simulink model "FEEDER_MODEL"  (R2024b)
settings: Solver=ode23t  StartTime=0.0  StopTime=2.4  RelTol=1e-3
libraries: spsFirstOrderFilterLib x42, spsThreePhaseVIMeasurementLib x7, spsThreePhaseDynamicLoadLib x4, spsDistributedParametersLineLib x4, spsPower3phInstantaneousLib x3, spsThreePhaseSourceLib x2, spsThreePhaseTransformerTwoWindingsLib x2, spspowerguiLib x1
(part 2 of 2)

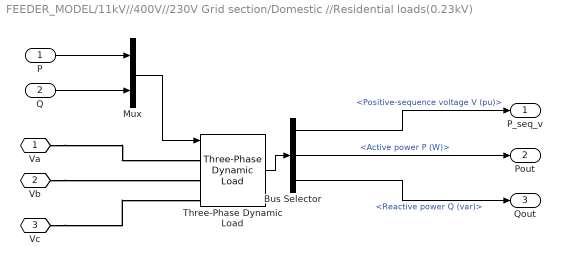
== system FEEDER_MODEL/11kV//400V//230V Grid section/Domestic //Residential loads(0.23kV) ==
  P : Inport
  Q : Inport  Port=2
  Bus Selector : BusSelector  OutputSignals=Positive-sequence voltage V (pu),Active power P (W),Reactive power Q (var)
  Mux : Mux  Inputs=2
  Three-Phase Dynamic Load : spsThreePhaseDynamicLoadLib/Three-Phase Dynamic Load  NominalVoltage=[ 230 50 ]  ActiveReactivePowers=[5e3 3.1e3]  PositiveSequence=[0.994 -11.8]  ExternalControl=on  NpNq=[1.3 2]  TimeConstants="[0  0  0  0]"  MinimumVoltage=0.7  Tfilter=1e-4  LoadFlowParameters=[4,0,0,0,0]
  Va : PMIOPort  Side=Left
  Vb : PMIOPort  Port=2  Side=Left
  Vc : PMIOPort  Port=3  Side=Left
  P_seq_v : Outport
  Pout : Outport  Port=2
  Qout : Outport  Port=3
  wires:
  Bus Selector/1 -> P_seq_v/1  "<Positive-sequence voltage V (pu)>"
  P/1 -> Mux/1
  Q/1 -> Mux/2
  Three-Phase Dynamic Load/1 -> Bus Selector/1
  Bus Selector/2 -> Pout/1  "<Active power P (W)>"
  Mux/1 -> Three-Phase Dynamic Load/1
  Bus Selector/3 -> Qout/1  "<Reactive power Q (var)>"
  connections:
  Va/RConn1 -- Three-Phase Dynamic Load/LConn1
  Vb/RConn1 -- Three-Phase Dynamic Load/LConn2
  Vc/RConn1 -- Three-Phase Dynamic Load/LConn3

== system FEEDER_MODEL/11kV//400V//230V Grid section/Filter1 ==
  Signal_in : Inport
  First-Order Filter18 : spsFirstOrderFilterLib/First-Order Filter  FilterType=Lowpass  Tc=1/(2*pi*50)  Ts=0  Initialize=off  Vac_Init=[0, 0, 50]  Vdc_Init=0  PlotResponse=off  FreqRange="[0,  200,  1]"
  First-Order Filter19 : spsFirstOrderFilterLib/First-Order Filter  FilterType=Lowpass  Tc=1/(2*pi*50)  Ts=0  Initialize=off  Vac_Init=[0, 0, 50]  Vdc_Init=0  PlotResponse=off  FreqRange="[0,  200,  1]"
  First-Order Filter20 : spsFirstOrderFilterLib/First-Order Filter  FilterType=Lowpass  Tc=1/(2*pi*50)  Ts=0  Initialize=off  Vac_Init=[0, 0, 50]  Vdc_Init=0  PlotResponse=off  FreqRange="[0,  200,  1]"
  F_Signal_out : Outport
  wires:
  First-Order Filter18/1 -> First-Order Filter19/1
  First-Order Filter20/1 -> F_Signal_out/1
  First-Order Filter19/1 -> First-Order Filter20/1
  Signal_in/1 -> First-Order Filter18/1

== system FEEDER_MODEL/11kV//400V//230V Grid section/Filter10 ==
  Signal_in : Inport
  First-Order Filter18 : spsFirstOrderFilterLib/First-Order Filter  FilterType=Lowpass  Tc=1/(2*pi*50)  Ts=0  Initialize=off  Vac_Init=[0, 0, 50]  Vdc_Init=0  PlotResponse=off  FreqRange="[0,  200,  1]"
  First-Order Filter19 : spsFirstOrderFilterLib/First-Order Filter  FilterType=Lowpass  Tc=1/(2*pi*50)  Ts=0  Initialize=off  Vac_Init=[0, 0, 50]  Vdc_Init=0  PlotResponse=off  FreqRange="[0,  200,  1]"
  First-Order Filter20 : spsFirstOrderFilterLib/First-Order Filter  FilterType=Lowpass  Tc=1/(2*pi*50)  Ts=0  Initialize=off  Vac_Init=[0, 0, 50]  Vdc_Init=0  PlotResponse=off  FreqRange="[0,  200,  1]"
  F_Signal_out : Outport
  wires:
  Signal_in/1 -> First-Order Filter18/1
  First-Order Filter19/1 -> First-Order Filter20/1
  First-Order Filter20/1 -> F_Signal_out/1
  First-Order Filter18/1 -> First-Order Filter19/1

== system FEEDER_MODEL/11kV//400V//230V Grid section/Filter11 ==
  Signal_in : Inport
  First-Order Filter18 : spsFirstOrderFilterLib/First-Order Filter  FilterType=Lowpass  Tc=1/(2*pi*50)  Ts=0  Initialize=off  Vac_Init=[0, 0, 50]  Vdc_Init=0  PlotResponse=off  FreqRange="[0,  200,  1]"
  First-Order Filter19 : spsFirstOrderFilterLib/First-Order Filter  FilterType=Lowpass  Tc=1/(2*pi*50)  Ts=0  Initialize=off  Vac_Init=[0, 0, 50]  Vdc_Init=0  PlotResponse=off  FreqRange="[0,  200,  1]"
  First-Order Filter20 : spsFirstOrderFilterLib/First-Order Filter  FilterType=Lowpass  Tc=1/(2*pi*50)  Ts=0  Initialize=off  Vac_Init=[0, 0, 50]  Vdc_Init=0  PlotResponse=off  FreqRange="[0,  200,  1]"
  F_Signal_out : Outport
  wires:
  First-Order Filter18/1 -> First-Order Filter19/1
  First-Order Filter20/1 -> F_Signal_out/1
  First-Order Filter19/1 -> First-Order Filter20/1
  Signal_in/1 -> First-Order Filter18/1

== system FEEDER_MODEL/11kV//400V//230V Grid section/Filter12 ==
  Signal_in : Inport
  First-Order Filter18 : spsFirstOrderFilterLib/First-Order Filter  FilterType=Lowpass  Tc=1/(2*pi*50)  Ts=0  Initialize=off  Vac_Init=[0, 0, 50]  Vdc_Init=0  PlotResponse=off  FreqRange="[0,  200,  1]"
  First-Order Filter19 : spsFirstOrderFilterLib/First-Order Filter  FilterType=Lowpass  Tc=1/(2*pi*50)  Ts=0  Initialize=off  Vac_Init=[0, 0, 50]  Vdc_Init=0  PlotResponse=off  FreqRange="[0,  200,  1]"
  First-Order Filter20 : spsFirstOrderFilterLib/First-Order Filter  FilterType=Lowpass  Tc=1/(2*pi*50)  Ts=0  Initialize=off  Vac_Init=[0, 0, 50]  Vdc_Init=0  PlotResponse=off  FreqRange="[0,  200,  1]"
  F_Signal_out : Outport
  wires:
  Signal_in/1 -> First-Order Filter18/1
  First-Order Filter19/1 -> First-Order Filter20/1
  First-Order Filter20/1 -> F_Signal_out/1
  First-Order Filter18/1 -> First-Order Filter19/1

== system FEEDER_MODEL/11kV//400V//230V Grid section/Filter13 ==
  Signal_in : Inport
  First-Order Filter18 : spsFirstOrderFilterLib/First-Order Filter  FilterType=Lowpass  Tc=1/(2*pi*50)  Ts=0  Initialize=off  Vac_Init=[0, 0, 50]  Vdc_Init=0  PlotResponse=off  FreqRange="[0,  200,  1]"
  First-Order Filter19 : spsFirstOrderFilterLib/First-Order Filter  FilterType=Lowpass  Tc=1/(2*pi*50)  Ts=0  Initialize=off  Vac_Init=[0, 0, 50]  Vdc_Init=0  PlotResponse=off  FreqRange="[0,  200,  1]"
  First-Order Filter20 : spsFirstOrderFilterLib/First-Order Filter  FilterType=Lowpass  Tc=1/(2*pi*50)  Ts=0  Initialize=off  Vac_Init=[0, 0, 50]  Vdc_Init=0  PlotResponse=off  FreqRange="[0,  200,  1]"
  F_Signal_out : Outport
  wires:
  First-Order Filter18/1 -> First-Order Filter19/1
  First-Order Filter20/1 -> F_Signal_out/1
  First-Order Filter19/1 -> First-Order Filter20/1
  Signal_in/1 -> First-Order Filter18/1

== system FEEDER_MODEL/11kV//400V//230V Grid section/Filter14 ==
  Signal_in : Inport
  First-Order Filter18 : spsFirstOrderFilterLib/First-Order Filter  FilterType=Lowpass  Tc=1/(2*pi*50)  Ts=0  Initialize=off  Vac_Init=[0, 0, 50]  Vdc_Init=0  PlotResponse=off  FreqRange="[0,  200,  1]"
  First-Order Filter19 : spsFirstOrderFilterLib/First-Order Filter  FilterType=Lowpass  Tc=1/(2*pi*50)  Ts=0  Initialize=off  Vac_Init=[0, 0, 50]  Vdc_Init=0  PlotResponse=off  FreqRange="[0,  200,  1]"
  First-Order Filter20 : spsFirstOrderFilterLib/First-Order Filter  FilterType=Lowpass  Tc=1/(2*pi*50)  Ts=0  Initialize=off  Vac_Init=[0, 0, 50]  Vdc_Init=0  PlotResponse=off  FreqRange="[0,  200,  1]"
  F_Signal_out : Outport
  wires:
  Signal_in/1 -> First-Order Filter18/1
  First-Order Filter19/1 -> First-Order Filter20/1
  First-Order Filter20/1 -> F_Signal_out/1
  First-Order Filter18/1 -> First-Order Filter19/1

== system FEEDER_MODEL/11kV//400V//230V Grid section/Filter2 ==
  Signal_in : Inport
  First-Order Filter18 : spsFirstOrderFilterLib/First-Order Filter  FilterType=Lowpass  Tc=1/(2*pi*50)  Ts=0  Initialize=off  Vac_Init=[0, 0, 50]  Vdc_Init=0  PlotResponse=off  FreqRange="[0,  200,  1]"
  First-Order Filter19 : spsFirstOrderFilterLib/First-Order Filter  FilterType=Lowpass  Tc=1/(2*pi*50)  Ts=0  Initialize=off  Vac_Init=[0, 0, 50]  Vdc_Init=0  PlotResponse=off  FreqRange="[0,  200,  1]"
  First-Order Filter20 : spsFirstOrderFilterLib/First-Order Filter  FilterType=Lowpass  Tc=1/(2*pi*50)  Ts=0  Initialize=off  Vac_Init=[0, 0, 50]  Vdc_Init=0  PlotResponse=off  FreqRange="[0,  200,  1]"
  F_Signal_out : Outport
  wires:
  Signal_in/1 -> First-Order Filter18/1
  First-Order Filter19/1 -> First-Order Filter20/1
  First-Order Filter20/1 -> F_Signal_out/1
  First-Order Filter18/1 -> First-Order Filter19/1

== system FEEDER_MODEL/11kV//400V//230V Grid section/Filter3 ==
  Signal_in : Inport
  First-Order Filter18 : spsFirstOrderFilterLib/First-Order Filter  FilterType=Lowpass  Tc=1/(2*pi*50)  Ts=0  Initialize=off  Vac_Init=[0, 0, 50]  Vdc_Init=0  PlotResponse=off  FreqRange="[0,  200,  1]"
  First-Order Filter19 : spsFirstOrderFilterLib/First-Order Filter  FilterType=Lowpass  Tc=1/(2*pi*50)  Ts=0  Initialize=off  Vac_Init=[0, 0, 50]  Vdc_Init=0  PlotResponse=off  FreqRange="[0,  200,  1]"
  First-Order Filter20 : spsFirstOrderFilterLib/First-Order Filter  FilterType=Lowpass  Tc=1/(2*pi*50)  Ts=0  Initialize=off  Vac_Init=[0, 0, 50]  Vdc_Init=0  PlotResponse=off  FreqRange="[0,  200,  1]"
  F_Signal_out : Outport
  wires:
  Signal_in/1 -> First-Order Filter18/1
  First-Order Filter19/1 -> First-Order Filter20/1
  First-Order Filter20/1 -> F_Signal_out/1
  First-Order Filter18/1 -> First-Order Filter19/1

== system FEEDER_MODEL/11kV//400V//230V Grid section/Filter4 ==
  Signal_in : Inport
  First-Order Filter18 : spsFirstOrderFilterLib/First-Order Filter  FilterType=Lowpass  Tc=1/(2*pi*50)  Ts=0  Initialize=off  Vac_Init=[0, 0, 50]  Vdc_Init=0  PlotResponse=off  FreqRange="[0,  200,  1]"
  First-Order Filter19 : spsFirstOrderFilterLib/First-Order Filter  FilterType=Lowpass  Tc=1/(2*pi*50)  Ts=0  Initialize=off  Vac_Init=[0, 0, 50]  Vdc_Init=0  PlotResponse=off  FreqRange="[0,  200,  1]"
  First-Order Filter20 : spsFirstOrderFilterLib/First-Order Filter  FilterType=Lowpass  Tc=1/(2*pi*50)  Ts=0  Initialize=off  Vac_Init=[0, 0, 50]  Vdc_Init=0  PlotResponse=off  FreqRange="[0,  200,  1]"
  F_Signal_out : Outport
  wires:
  Signal_in/1 -> First-Order Filter18/1
  First-Order Filter19/1 -> First-Order Filter20/1
  First-Order Filter20/1 -> F_Signal_out/1
  First-Order Filter18/1 -> First-Order Filter19/1

== system FEEDER_MODEL/11kV//400V//230V Grid section/Filter5 ==
  Signal_in : Inport
  First-Order Filter18 : spsFirstOrderFilterLib/First-Order Filter  FilterType=Lowpass  Tc=1/(2*pi*50)  Ts=0  Initialize=off  Vac_Init=[0, 0, 50]  Vdc_Init=0  PlotResponse=off  FreqRange="[0,  200,  1]"
  First-Order Filter19 : spsFirstOrderFilterLib/First-Order Filter  FilterType=Lowpass  Tc=1/(2*pi*50)  Ts=0  Initialize=off  Vac_Init=[0, 0, 50]  Vdc_Init=0  PlotResponse=off  FreqRange="[0,  200,  1]"
  First-Order Filter20 : spsFirstOrderFilterLib/First-Order Filter  FilterType=Lowpass  Tc=1/(2*pi*50)  Ts=0  Initialize=off  Vac_Init=[0, 0, 50]  Vdc_Init=0  PlotResponse=off  FreqRange="[0,  200,  1]"
  F_Signal_out : Outport
  wires:
  First-Order Filter18/1 -> First-Order Filter19/1
  First-Order Filter20/1 -> F_Signal_out/1
  First-Order Filter19/1 -> First-Order Filter20/1
  Signal_in/1 -> First-Order Filter18/1

== system FEEDER_MODEL/11kV//400V//230V Grid section/Filter6 ==
  Signal_in : Inport
  First-Order Filter18 : spsFirstOrderFilterLib/First-Order Filter  FilterType=Lowpass  Tc=1/(2*pi*50)  Ts=0  Initialize=off  Vac_Init=[0, 0, 50]  Vdc_Init=0  PlotResponse=off  FreqRange="[0,  200,  1]"
  First-Order Filter19 : spsFirstOrderFilterLib/First-Order Filter  FilterType=Lowpass  Tc=1/(2*pi*50)  Ts=0  Initialize=off  Vac_Init=[0, 0, 50]  Vdc_Init=0  PlotResponse=off  FreqRange="[0,  200,  1]"
  First-Order Filter20 : spsFirstOrderFilterLib/First-Order Filter  FilterType=Lowpass  Tc=1/(2*pi*50)  Ts=0  Initialize=off  Vac_Init=[0, 0, 50]  Vdc_Init=0  PlotResponse=off  FreqRange="[0,  200,  1]"
  F_Signal_out : Outport
  wires:
  Signal_in/1 -> First-Order Filter18/1
  First-Order Filter19/1 -> First-Order Filter20/1
  First-Order Filter20/1 -> F_Signal_out/1
  First-Order Filter18/1 -> First-Order Filter19/1

== system FEEDER_MODEL/11kV//400V//230V Grid section/Filter7 ==
  Signal_in : Inport
  First-Order Filter18 : spsFirstOrderFilterLib/First-Order Filter  FilterType=Lowpass  Tc=1/(2*pi*50)  Ts=0  Initialize=off  Vac_Init=[0, 0, 50]  Vdc_Init=0  PlotResponse=off  FreqRange="[0,  200,  1]"
  First-Order Filter19 : spsFirstOrderFilterLib/First-Order Filter  FilterType=Lowpass  Tc=1/(2*pi*50)  Ts=0  Initialize=off  Vac_Init=[0, 0, 50]  Vdc_Init=0  PlotResponse=off  FreqRange="[0,  200,  1]"
  First-Order Filter20 : spsFirstOrderFilterLib/First-Order Filter  FilterType=Lowpass  Tc=1/(2*pi*50)  Ts=0  Initialize=off  Vac_Init=[0, 0, 50]  Vdc_Init=0  PlotResponse=off  FreqRange="[0,  200,  1]"
  F_Signal_out : Outport
  wires:
  First-Order Filter18/1 -> First-Order Filter19/1
  First-Order Filter20/1 -> F_Signal_out/1
  First-Order Filter19/1 -> First-Order Filter20/1
  Signal_in/1 -> First-Order Filter18/1

== system FEEDER_MODEL/11kV//400V//230V Grid section/Filter8 ==
  Signal_in : Inport
  First-Order Filter18 : spsFirstOrderFilterLib/First-Order Filter  FilterType=Lowpass  Tc=1/(2*pi*50)  Ts=0  Initialize=off  Vac_Init=[0, 0, 50]  Vdc_Init=0  PlotResponse=off  FreqRange="[0,  200,  1]"
  First-Order Filter19 : spsFirstOrderFilterLib/First-Order Filter  FilterType=Lowpass  Tc=1/(2*pi*50)  Ts=0  Initialize=off  Vac_Init=[0, 0, 50]  Vdc_Init=0  PlotResponse=off  FreqRange="[0,  200,  1]"
  First-Order Filter20 : spsFirstOrderFilterLib/First-Order Filter  FilterType=Lowpass  Tc=1/(2*pi*50)  Ts=0  Initialize=off  Vac_Init=[0, 0, 50]  Vdc_Init=0  PlotResponse=off  FreqRange="[0,  200,  1]"
  F_Signal_out : Outport
  wires:
  First-Order Filter18/1 -> First-Order Filter19/1
  First-Order Filter20/1 -> F_Signal_out/1
  First-Order Filter19/1 -> First-Order Filter20/1
  Signal_in/1 -> First-Order Filter18/1

== system FEEDER_MODEL/11kV//400V//230V Grid section/Filter9 ==
  Signal_in : Inport
  First-Order Filter18 : spsFirstOrderFilterLib/First-Order Filter  FilterType=Lowpass  Tc=1/(2*pi*50)  Ts=0  Initialize=off  Vac_Init=[0, 0, 50]  Vdc_Init=0  PlotResponse=off  FreqRange="[0,  200,  1]"
  First-Order Filter19 : spsFirstOrderFilterLib/First-Order Filter  FilterType=Lowpass  Tc=1/(2*pi*50)  Ts=0  Initialize=off  Vac_Init=[0, 0, 50]  Vdc_Init=0  PlotResponse=off  FreqRange="[0,  200,  1]"
  First-Order Filter20 : spsFirstOrderFilterLib/First-Order Filter  FilterType=Lowpass  Tc=1/(2*pi*50)  Ts=0  Initialize=off  Vac_Init=[0, 0, 50]  Vdc_Init=0  PlotResponse=off  FreqRange="[0,  200,  1]"
  F_Signal_out : Outport
  wires:
  Signal_in/1 -> First-Order Filter18/1
  First-Order Filter19/1 -> First-Order Filter20/1
  First-Order Filter20/1 -> F_Signal_out/1
  First-Order Filter18/1 -> First-Order Filter19/1

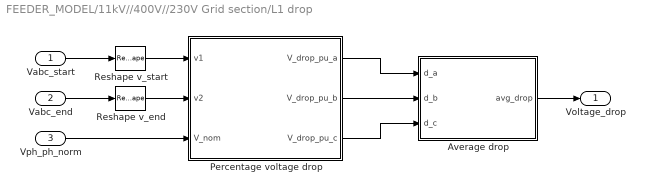
== system FEEDER_MODEL/11kV//400V//230V Grid section/L1 drop ==
  Vabc_start : Inport
  Vabc_end : Inport  Port=2
  Vph_ph_norm : Inport  Port=3
  Average drop : MATLAB Function  TreatAsAtomicUnit=on
  Percentage voltage drop : MATLAB Function  TreatAsAtomicUnit=on
  Reshape v_end : Reshape  OutputDimensionality=Customize  OutputDimensions=[3,1]
  Reshape v_start : Reshape  OutputDimensionality=Customize  OutputDimensions=[3,1]
  Voltage_drop : Outport
  wires:
  Reshape v_end/1 -> Percentage voltage drop/2(v2)
  Percentage voltage drop/3(V_drop_pu_c) -> Average drop/3(d_c)
  Vabc_start/1 -> Reshape v_start/1
  Reshape v_start/1 -> Percentage voltage drop/1(v1)
  Vph_ph_norm/1 -> Percentage voltage drop/3(V_nom)
  Percentage voltage drop/2(V_drop_pu_b) -> Average drop/2(d_b)
  Average drop/1(avg_drop) -> Voltage_drop/1
  Vabc_end/1 -> Reshape v_end/1
  Percentage voltage drop/1(V_drop_pu_a) -> Average drop/1(d_a)

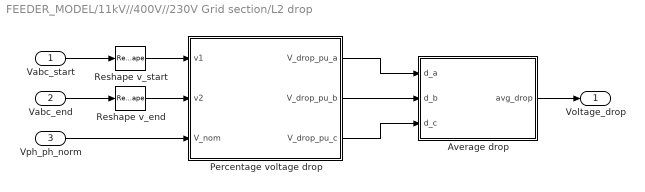
== system FEEDER_MODEL/11kV//400V//230V Grid section/L2 drop ==
  Vabc_start : Inport
  Vabc_end : Inport  Port=2
  Vph_ph_norm : Inport  Port=3
  Average drop : MATLAB Function  TreatAsAtomicUnit=on
  Percentage voltage drop : MATLAB Function  TreatAsAtomicUnit=on
  Reshape v_end : Reshape  OutputDimensionality=Customize  OutputDimensions=[3,1]
  Reshape v_start : Reshape  OutputDimensionality=Customize  OutputDimensions=[3,1]
  Voltage_drop : Outport
  wires:
  Percentage voltage drop/1(V_drop_pu_a) -> Average drop/1(d_a)
  Vabc_end/1 -> Reshape v_end/1
  Average drop/1(avg_drop) -> Voltage_drop/1
  Percentage voltage drop/2(V_drop_pu_b) -> Average drop/2(d_b)
  Vph_ph_norm/1 -> Percentage voltage drop/3(V_nom)
  Reshape v_start/1 -> Percentage voltage drop/1(v1)
  Vabc_start/1 -> Reshape v_start/1
  Percentage voltage drop/3(V_drop_pu_c) -> Average drop/3(d_c)
  Reshape v_end/1 -> Percentage voltage drop/2(v2)

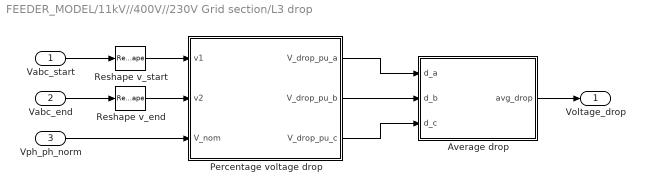
== system FEEDER_MODEL/11kV//400V//230V Grid section/L3 drop ==
  Vabc_start : Inport
  Vabc_end : Inport  Port=2
  Vph_ph_norm : Inport  Port=3
  Average drop : MATLAB Function  TreatAsAtomicUnit=on
  Percentage voltage drop : MATLAB Function  TreatAsAtomicUnit=on
  Reshape v_end : Reshape  OutputDimensionality=Customize  OutputDimensions=[3,1]
  Reshape v_start : Reshape  OutputDimensionality=Customize  OutputDimensions=[3,1]
  Voltage_drop : Outport
  wires:
  Reshape v_end/1 -> Percentage voltage drop/2(v2)
  Percentage voltage drop/3(V_drop_pu_c) -> Average drop/3(d_c)
  Vabc_start/1 -> Reshape v_start/1
  Reshape v_start/1 -> Percentage voltage drop/1(v1)
  Vph_ph_norm/1 -> Percentage voltage drop/3(V_nom)
  Percentage voltage drop/2(V_drop_pu_b) -> Average drop/2(d_b)
  Average drop/1(avg_drop) -> Voltage_drop/1
  Vabc_end/1 -> Reshape v_end/1
  Percentage voltage drop/1(V_drop_pu_a) -> Average drop/1(d_a)

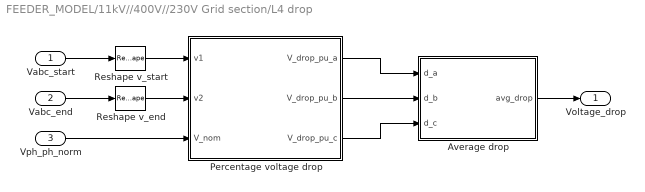
== system FEEDER_MODEL/11kV//400V//230V Grid section/L4 drop ==
  Vabc_start : Inport
  Vabc_end : Inport  Port=2
  Vph_ph_norm : Inport  Port=3
  Average drop : MATLAB Function  TreatAsAtomicUnit=on
  Percentage voltage drop : MATLAB Function  TreatAsAtomicUnit=on
  Reshape v_end : Reshape  OutputDimensionality=Customize  OutputDimensions=[3,1]
  Reshape v_start : Reshape  OutputDimensionality=Customize  OutputDimensions=[3,1]
  Voltage_drop : Outport
  wires:
  Percentage voltage drop/1(V_drop_pu_a) -> Average drop/1(d_a)
  Vabc_end/1 -> Reshape v_end/1
  Average drop/1(avg_drop) -> Voltage_drop/1
  Percentage voltage drop/2(V_drop_pu_b) -> Average drop/2(d_b)
  Vph_ph_norm/1 -> Percentage voltage drop/3(V_nom)
  Reshape v_start/1 -> Percentage voltage drop/1(v1)
  Vabc_start/1 -> Reshape v_start/1
  Percentage voltage drop/3(V_drop_pu_c) -> Average drop/3(d_c)
  Reshape v_end/1 -> Percentage voltage drop/2(v2)

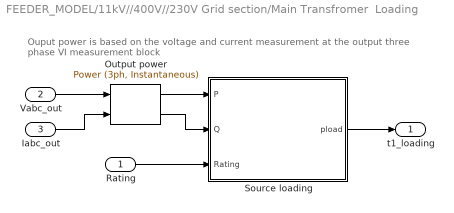
== system FEEDER_MODEL/11kV//400V//230V Grid section/Main Transfromer  Loading ==
  note: Ouput power is based on the voltage and current measurement at the output three
      | phase VI measurement block
  Rating : Inport
  Vabc_out : Inport  Port=2
  Iabc_out : Inport  Port=3
  Output power : spsPower3phInstantaneousLib/Power (3ph, Instantaneous)
  Source loading : MATLAB Function  TreatAsAtomicUnit=on
  t1_loading : Outport
  wires:
  Output power/2 -> Source loading/2(Q)
  Output power/1 -> Source loading/1(P)
  Source loading/1(pload) -> t1_loading/1
  Vabc_out/1 -> Output power/1
  Iabc_out/1 -> Output power/2
  Rating/1 -> Source loading/3(Rating)

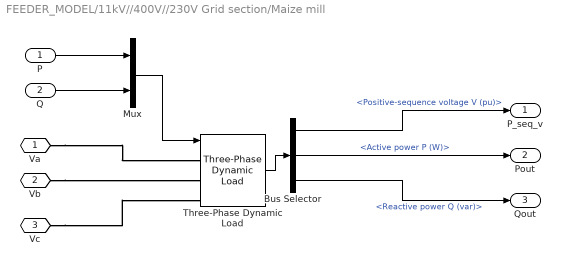
== system FEEDER_MODEL/11kV//400V//230V Grid section/Maize mill ==
  P : Inport
  Q : Inport  Port=2
  Bus Selector : BusSelector  OutputSignals=Positive-sequence voltage V (pu),Active power P (W),Reactive power Q (var)
  Mux : Mux  Inputs=2
  Three-Phase Dynamic Load : spsThreePhaseDynamicLoadLib/Three-Phase Dynamic Load  NominalVoltage=[ 400 50 ]  ActiveReactivePowers=[1e3 6.2e2]  PositiveSequence=[0.994 -11.8]  ExternalControl=on  NpNq=[1.3 2]  TimeConstants="[0  0  0  0]"  MinimumVoltage=0.7  Tfilter=1e-4  LoadFlowParameters=[4,0,0,0,0]
  Va : PMIOPort  Side=Left
  Vb : PMIOPort  Port=2  Side=Left
  Vc : PMIOPort  Port=3  Side=Left
  P_seq_v : Outport
  Pout : Outport  Port=2
  Qout : Outport  Port=3
  wires:
  Bus Selector/1 -> P_seq_v/1  "<Positive-sequence voltage V (pu)>"
  P/1 -> Mux/1
  Q/1 -> Mux/2
  Three-Phase Dynamic Load/1 -> Bus Selector/1
  Bus Selector/2 -> Pout/1  "<Active power P (W)>"
  Mux/1 -> Three-Phase Dynamic Load/1
  Bus Selector/3 -> Qout/1  "<Reactive power Q (var)>"
  connections:
  Va/RConn1 -- Three-Phase Dynamic Load/LConn1
  Vb/RConn1 -- Three-Phase Dynamic Load/LConn2
  Vc/RConn1 -- Three-Phase Dynamic Load/LConn3

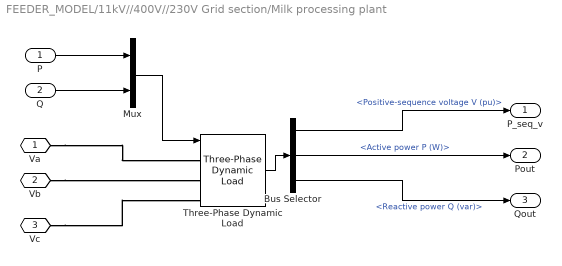
== system FEEDER_MODEL/11kV//400V//230V Grid section/Milk processing plant ==
  P : Inport
  Q : Inport  Port=2
  Bus Selector : BusSelector  OutputSignals=Positive-sequence voltage V (pu),Active power P (W),Reactive power Q (var)
  Mux : Mux  Inputs=2
  Three-Phase Dynamic Load : spsThreePhaseDynamicLoadLib/Three-Phase Dynamic Load  NominalVoltage=[ 400 50 ]  ActiveReactivePowers=[5e3 3.1e3]  PositiveSequence=[0.994 -11.8]  ExternalControl=on  NpNq=[1.3 2]  TimeConstants="[0  0  0  0]"  MinimumVoltage=0.7  Tfilter=1e-4  LoadFlowParameters=[4,0,0,0,0]
  Va : PMIOPort  Side=Left
  Vb : PMIOPort  Port=2  Side=Left
  Vc : PMIOPort  Port=3  Side=Left
  P_seq_v : Outport
  Pout : Outport  Port=2
  Qout : Outport  Port=3
  wires:
  Bus Selector/3 -> Qout/1  "<Reactive power Q (var)>"
  Mux/1 -> Three-Phase Dynamic Load/1
  Bus Selector/2 -> Pout/1  "<Active power P (W)>"
  Three-Phase Dynamic Load/1 -> Bus Selector/1
  Q/1 -> Mux/2
  P/1 -> Mux/1
  Bus Selector/1 -> P_seq_v/1  "<Positive-sequence voltage V (pu)>"
  connections:
  Vc/RConn1 -- Three-Phase Dynamic Load/LConn3
  Vb/RConn1 -- Three-Phase Dynamic Load/LConn2
  Va/RConn1 -- Three-Phase Dynamic Load/LConn1

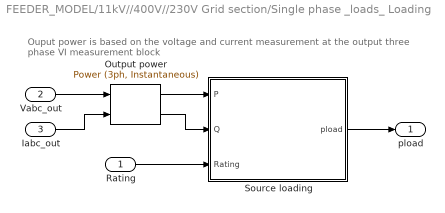
== system FEEDER_MODEL/11kV//400V//230V Grid section/Single phase _loads_ Loading ==
  note: Ouput power is based on the voltage and current measurement at the output three
      | phase VI measurement block
  Rating : Inport
  Vabc_out : Inport  Port=2
  Iabc_out : Inport  Port=3
  Output power : spsPower3phInstantaneousLib/Power (3ph, Instantaneous)
  Source loading : MATLAB Function  TreatAsAtomicUnit=on
  pload : Outport
  wires:
  Rating/1 -> Source loading/3(Rating)
  Iabc_out/1 -> Output power/2
  Vabc_out/1 -> Output power/1
  Source loading/1(pload) -> pload/1
  Output power/1 -> Source loading/1(P)
  Output power/2 -> Source loading/2(Q)

== system FEEDER_MODEL/11kV//400V//230V Grid section/Solar infeed power ==
  Vin : Inport
  Iin : Inport  Port=2
  Power infeed : spsPower3phInstantaneousLib/Power (3ph, Instantaneous)
  Inv_A : Outport
  Inv_R : Outport  Port=2
  wires:
  Power infeed/2 -> Inv_R/1
  Vin/1 -> Power infeed/1
  Iin/1 -> Power infeed/2
  Power infeed/1 -> Inv_A/1

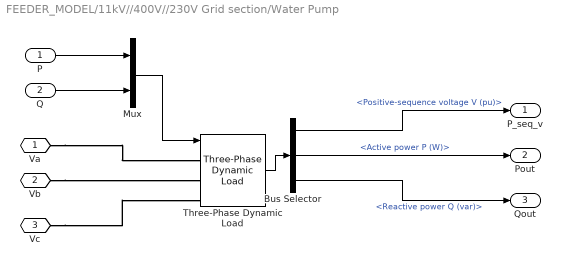
== system FEEDER_MODEL/11kV//400V//230V Grid section/Water Pump ==
  P : Inport
  Q : Inport  Port=2
  Bus Selector : BusSelector  OutputSignals=Positive-sequence voltage V (pu),Active power P (W),Reactive power Q (var)
  Mux : Mux  Inputs=2
  Three-Phase Dynamic Load : spsThreePhaseDynamicLoadLib/Three-Phase Dynamic Load  NominalVoltage=[ 400 50 ]  ActiveReactivePowers=[5e2 3.1e2]  PositiveSequence=[0.994 -11.8]  ExternalControl=on  NpNq=[1.3 2]  TimeConstants="[0  0  0  0]"  MinimumVoltage=0.7  Tfilter=1e-4  LoadFlowParameters=[4,0,0,0,0]
  Va : PMIOPort  Side=Left
  Vb : PMIOPort  Port=2  Side=Left
  Vc : PMIOPort  Port=3  Side=Left
  P_seq_v : Outport
  Pout : Outport  Port=2
  Qout : Outport  Port=3
  wires:
  Bus Selector/1 -> P_seq_v/1  "<Positive-sequence voltage V (pu)>"
  P/1 -> Mux/1
  Q/1 -> Mux/2
  Three-Phase Dynamic Load/1 -> Bus Selector/1
  Bus Selector/2 -> Pout/1  "<Active power P (W)>"
  Mux/1 -> Three-Phase Dynamic Load/1
  Bus Selector/3 -> Qout/1  "<Reactive power Q (var)>"
  connections:
  Va/RConn1 -- Three-Phase Dynamic Load/LConn1
  Vb/RConn1 -- Three-Phase Dynamic Load/LConn2
  Vc/RConn1 -- Three-Phase Dynamic Load/LConn3

== matlab function FEEDER_MODEL/11kV//400V//230V Grid section/L4 drop/Average drop ==
  data: d_a input; avg_drop output; d_b input; d_c input
function avg_drop = fcn(d_a,d_b,d_c)

avg_drop = ((d_a+d_b+d_c)/3)*100;
end

== matlab function FEEDER_MODEL/11kV//400V//230V Grid section/L1 drop/Average drop ==
  data: d_a input; avg_drop output; d_b input; d_c input
function avg_drop = fcn(d_a,d_b,d_c)

avg_drop = ((d_a+d_b+d_c)/3)*100;
end

== matlab function FEEDER_MODEL/11kV//400V//230V Grid section/L4 drop/Percentage voltage drop ==
  data: v1 input; V_drop_pu_a output; v2 input; V_drop_pu_b output; V_drop_pu_c output; V_nom input
function [V_drop_pu_a, V_drop_pu_b, V_drop_pu_c] = vdrop_pu(v1, v2, V_nom)
           % Input validation: Ensure inputs are 3x1 vectors
           if ~isequal(size(v1), [3,1]) || ~isequal(size(v2), [3,1])
               error('Inputs must be 3x1 vectors');
           end
           
           % Compute element-wise differences (voltage drops)
           diff = v1 - v2;
           
           % Compute per-unit voltage drops
           V_drop_pu_a = abs(diff(1)) / V_nom; % Per-unit voltage drop for phase a
           V_drop_pu_b = abs(diff(2)) / V_nom; % Per-unit voltage drop for phase b
           V_drop_pu_c = abs(diff(3)) / V_nom; % Per-unit voltage drop for phase c
       end

== matlab function FEEDER_MODEL/11kV//400V//230V Grid section/Average voltage drop ==
  data: a input; avg output; b input; c input; d input
function avg = avg_drop(a,b,c,d)

avg=(a+b+c+d)/3;
end

== matlab function FEEDER_MODEL/11kV//400V//230V Grid section/Water pump Apparent Power ==
  data: P input; S output; Q input
function S = A_Power(P,Q)

S=sqrt(P^2+Q^2);
end

== matlab function FEEDER_MODEL/11kV//400V//230V Grid section/Maize mill apparent power ==
  data: P input; S output; Q input
function S = A_Power(P,Q)

S=sqrt(P^2+Q^2);
end

== matlab function FEEDER_MODEL/11kV//400V//230V Grid section/Total system apparent power ==
  data: S1 input; s_total output; S2 input; S3 input; S4 input
function s_total =Total_S(S1,S2,S3,S4)

s_total = S1+S2+S3+S4;
end

== matlab function FEEDER_MODEL/11kV//400V//230V Grid section/Total active power ==
  data: P1 input; p_total output; P2 input; P3 input; P4 input
function p_total =Total_P(P1,P2,P3,P4)

p_total = P1+P2+P3+P4;
end

== matlab function FEEDER_MODEL/11kV//400V//230V Grid section/Total reactive power ==
  data: Q1 input; q_total output; Q2 input; Q3 input; Q4 input
function q_total =Total_Q(Q1,Q2,Q3,Q4)

q_total = Q1+Q2+Q3+Q4;
end

== matlab function FEEDER_MODEL/11kV//400V//230V Grid section/System power factor ==
  data: Total_P input; pf output; Total_S input
function pf = PowerFactor(Total_P,Total_S)

pf = Total_P/Total_S;
end

== matlab function FEEDER_MODEL/11kV//400V//230V Grid section/Water pump power factor ==
  data: Total_P input; pf output; Total_S input
function pf = PowerFactor(Total_P,Total_S)

pf = Total_P/Total_S;
end

== matlab function FEEDER_MODEL/11kV//400V//230V Grid section/Milking machine pf ==
  data: Total_P input; pf output; Total_S input
function pf = PowerFactor(Total_P,Total_S)

pf = Total_P/Total_S;
end

== matlab function FEEDER_MODEL/11kV//400V//230V Grid section/L1 drop/Percentage voltage drop ==
  data: v1 input; V_drop_pu_a output; v2 input; V_drop_pu_b output; V_drop_pu_c output; V_nom input
function [V_drop_pu_a, V_drop_pu_b, V_drop_pu_c] = vdrop_pu(v1, v2, V_nom)
           % Input validation: Ensuring inputs are 3x1 vectors
           if ~isequal(size(v1), [3,1]) || ~isequal(size(v2), [3,1])
               error('Inputs must be 3x1 vectors');
           end
           
           % Computing element-wise differences (voltage drops)
           diff = v1 - v2;
           
           % Computing per-unit voltage drops
           V_drop_pu_a = abs(diff(1)) / V_nom; % Per-unit voltage drop for phase a
           V_drop_pu_b = abs(diff(2)) / V_nom; % Per-unit voltage drop for phase b
           V_drop_pu_c = abs(diff(3)) / V_nom; % Per-unit voltage drop for phase c
       end

== matlab function FEEDER_MODEL/11kV//400V//230V Grid section/Miaze mill pf ==
  data: Total_P input; pf output; Total_S input
function pf = PowerFactor(Total_P,Total_S)

pf = Total_P/Total_S;
end

== matlab function FEEDER_MODEL/11kV//400V//230V Grid section/Domestic loads pf ==
  data: Total_P input; pf output; Total_S input
function pf = PowerFactor(Total_P,Total_S)

pf = Total_P/Total_S;
end

== matlab function FEEDER_MODEL/11kV//400V//230V Grid section/Solar infeed Apparent power ==
  data: P input; S output; Q input
function S = A_Power(P,Q)

S=sqrt(P^2+Q^2);
end

== matlab function FEEDER_MODEL/11kV//400V//230V Grid section/Solar supply power factor ==
  data: Total_P input; pf output; Total_S input
function pf = PowerFactor(Total_P,Total_S)

pf = Total_P/Total_S;
end

== matlab function FEEDER_MODEL/11kV//400V//230V Grid section/L2 drop/Average drop ==
  data: d_a input; avg_drop output; d_b input; d_c input
function avg_drop = fcn(d_a,d_b,d_c)

avg_drop = ((d_a+d_b+d_c)/3)*100;
end

== matlab function FEEDER_MODEL/11kV//400V//230V Grid section/L2 drop/Percentage voltage drop ==
  data: v1 input; V_drop_pu_a output; v2 input; V_drop_pu_b output; V_drop_pu_c output; V_nom input
function [V_drop_pu_a, V_drop_pu_b, V_drop_pu_c] = vdrop_pu(v1, v2, V_nom)
           % Input validation: Ensure inputs are 3x1 vectors
           if ~isequal(size(v1), [3,1]) || ~isequal(size(v2), [3,1])
               error('Inputs must be 3x1 vectors');
           end
           
           % Compute element-wise differences (voltage drops)
           diff = v1 - v2;
           
           % Compute per-unit voltage drops
           V_drop_pu_a = abs(diff(1)) / V_nom; % Per-unit voltage drop for phase a
           V_drop_pu_b = abs(diff(2)) / V_nom; % Per-unit voltage drop for phase b
           V_drop_pu_c = abs(diff(3)) / V_nom; % Per-unit voltage drop for phase c
       end

== matlab function FEEDER_MODEL/11kV//400V//230V Grid section/L3 drop/Average drop ==
  data: d_a input; avg_drop output; d_b input; d_c input
function avg_drop = fcn(d_a,d_b,d_c)

avg_drop = ((d_a+d_b+d_c)/3)*100;
end

== matlab function FEEDER_MODEL/11kV//400V//230V Grid section/Main Transfromer  Loading/Source loading ==
  data: P input; pload output; Q input; Rating input
function pload = Loading(P,Q,Rating)

pload = ((sqrt(P^2+Q^2))/Rating)*100;
end

== matlab function FEEDER_MODEL/11kV//400V//230V Grid section/Milking machine apparent  power ==
  data: P input; S output; Q input
function S = A_Power(P,Q)

S=sqrt(P^2+Q^2);
end

== matlab function FEEDER_MODEL/11kV//400V//230V Grid section/Single phase _loads_ Loading/Source loading ==
  data: P input; pload output; Q input; Rating input
function pload = Loading(P,Q,Rating)

pload = ((sqrt(P^2+Q^2))/Rating)*100;
end

== matlab function FEEDER_MODEL/11kV//400V//230V Grid section/Domestic_loads ==
  data: P input; S output; Q input
function S = A_Power(P,Q)

S=sqrt(P^2+Q^2);
end

== matlab function FEEDER_MODEL/11kV//400V//230V Grid section/L3 drop/Percentage voltage drop ==
  data: v1 input; V_drop_pu_a output; v2 input; V_drop_pu_b output; V_drop_pu_c output; V_nom input
function [V_drop_pu_a, V_drop_pu_b, V_drop_pu_c] = vdrop_pu(v1, v2, V_nom)
           % Input validation: Ensure inputs are 3x1 vectors
           if ~isequal(size(v1), [3,1]) || ~isequal(size(v2), [3,1])
               error('Inputs must be 3x1 vectors');
           end
           
           % Compute element-wise differences (voltage drops)
           diff = v1 - v2;
           
           % Compute per-unit voltage drops
           V_drop_pu_a = abs(diff(1)) / V_nom; % Per-unit voltage drop for phase a
           V_drop_pu_b = abs(diff(2)) / V_nom; % Per-unit voltage drop for phase b
           V_drop_pu_c = abs(diff(3)) / V_nom; % Per-unit voltage drop for phase c
       end
